simulink model "EnablePort5"  (R2017b)
settings: Solver=FixedStepAuto  StartTime=0.0  StopTime=10.0  FixedStep=0.200000  RelTol=1e-3  EnableMultiTasking=on
settings Model: Creator=hbourbou  LastModifiedBy=hbourbou
settings DataIOCC: LimitDataPoints=on
settings OptimizationCC: LifeSpan=inf
settings DebuggingCC: SFUnexpectedBacktrackingDiag=warning  SFNoUnconditionalDefaultTransitionDiag=warning  SFExecutionAtInitializationDiag=none
settings HardwareCC: ProdBitPerSizeT=32  ProdBitPerPtrDiffT=32  ProdWordSize=32  ProdHWDeviceType=Specified
settings ModelReferenceCC: PropagateSignalLabelsOutOfModel=off
settings CodeAppCC: StateflowObjectComments=on
settings GRTTargetCC: TargetLangStandard=C89/C90 (ANSI)
settings ConfigComp: CovMetricSettings=dw  CovHtmlReporting=on  CovSaveCumulativeToWorkspaceVar=on  CovSaveSingleToWorkspaceVar=on  CovExternalEMLEnable=off

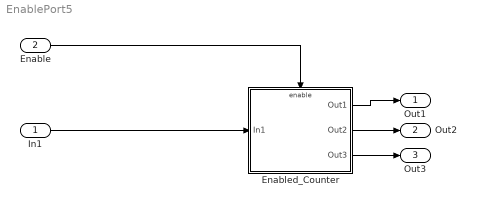
== system EnablePort5 ==
  In1 : Inport
  Enable : Inport  Port=2
  Enabled_Counter : Subsystem  TreatAsAtomicUnit=on
  Out1 : Outport
  Out2 : Outport  Port=2
  Out3 : Outport  Port=3
  wires:
  Enabled_Counter/1(Out1) -> Out1/1
  Enabled_Counter/2(Out2) -> Out2/1
  Enabled_Counter/3(Out3) -> Out3/1
  Enable/1 -> Enabled_Counter/Enable
  In1/1 -> Enabled_Counter/1(In1)

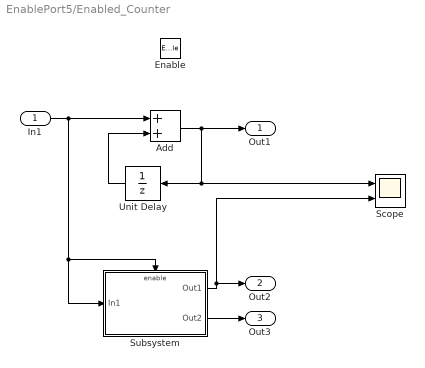
== system EnablePort5/Enabled_Counter ==
  In1 : Inport
  Enable : EnablePort
  Add : Sum
  Scope : Scope  NumInputPorts=2
  Subsystem : Subsystem  TreatAsAtomicUnit=on
  Unit Delay : UnitDelay  SampleTime=-1
  Out1 : Outport  InitialOutput=0
  Out2 : Outport  Port=2
  Out3 : Outport  Port=3
  wires:
  Unit Delay/1 -> Add/2
  Subsystem/1(Out1) -> Scope/2, Out2/1
  In1/1 -> Subsystem/Enable, Subsystem/1(In1), Add/1
  Add/1 -> Scope/1, Unit Delay/1, Out1/1
  Subsystem/2(Out2) -> Out3/1

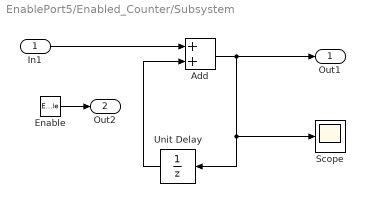
== system EnablePort5/Enabled_Counter/Subsystem ==
  In1 : Inport
  Enable : EnablePort  ShowOutputPort=on
  Add : Sum
  Scope : Scope
  Unit Delay : UnitDelay  SampleTime=-1
  Out1 : Outport
  Out2 : Outport  Port=2
  wires:
  In1/1 -> Add/1
  Unit Delay/1 -> Add/2
  Add/1 -> Scope/1, Unit Delay/1, Out1/1
  Enable/1 -> Out2/1
